simulink model "ACC_CC_model_best_2017aV1"  (Simulink 9.0)
settings: Solver=FixedStepAuto  StartTime=0.0  StopTime=1000  RelTol=1e-3
InitFcn:
  | step=0.001;%时间步长
  | run par.m
values from neighbouring files (symbols this model uses):
  ax_1 = Pop(i,1)    [IGPSO.m]
  ax_2 = Pop(i,2)    [IGPSO.m]
  ess_init_soc = 0.9    [IGPSO.m]
  ess_max_ah_cap = 5    [IGPSO.m]
  ess_r_chg = [0.001393 0.001393 0.001393 0.001393 0.001256 0.001172 0.001099 0.001074 0.001058 0.001066 0.0011 0.001161 0.001244 0.001327 0.001327]*3/5*32    [IGPSO.m]
  ess_r_dis = [0.004178 0.004178 0.004178 0.004178 0.003769 0.003517 0.003296 0.003222 0.003173 0.003197 0.0033 0.003483 0.003732 0.00398 0.00398]*3/5*32    [IGPSO.m]
  ess_soc = [0 0.2 0.25 0.3 0.35 0.4 0.45 0.5 0.55 0.6 0.65 0.7 0.75 0.8 1]    [IGPSO.m]
  ess_voc = [3.124 3.36 3.42 3.479 3.501 3.524 3.547 3.569 3.593 3.616 3.65 3.684 3.72 3.756 3.9]*3*32    [IGPSO.m]
  mc_eff_map = [0.43,0.49,0.58,0.66,0.73,0.70,0.73,0.66,0.58,0.49,0.43 ... (first row only)    [IGPSO.m]
  mc_map_spd = [0;1000;2000;3000;3500;4000;5000;6000;6500;7000;8000]*(2*pi)/60    [IGPSO.m]
  mc_map_trq = motorMAP(1,2:end)    [IGPSO.m]
  mc_max_trq = [142.2;148.6;146.5;92.4;83.9;71.1;56.9;48.4;43.4;37.7;35.6]    [IGPSO.m]
  v_base = 30    [IGPSO.m]
libraries: simulink x2, Solver_SF x1
(part 2 of 2)

== matlab function ACC-CC切换 ==
  data: d_logic1 output double; d_logic2 output double; u output double; vset input double; vp input double; v input double; d input double; d_des input double; lastmodel input double
function [ d_logic1,d_logic2,u]  = fcn(vset,vp,v,d,d_des,lastmodel)
% u=1：代表ACC   U=2代表CC
vset=vset/3.6;
vp=vp/3.6;
v=v/3.6;

k2=1.2;d1=2;
k1=1.999-1.196*exp(-0.1299*(vset-vp));
d_logic1=d_des+k1/2*(vset-vp)+k2*(v-vset)+d1;

k3=2;
d2=2;
k4=1.25;
d_logic2=d_des+k3*(vset-vp)+k4*(v-vp)+d2;

if vp>vset
    if d<d_des
        u=1;
    elseif (d>=d_des)&&(d<d_logic1)
        u=2;
    elseif (d>=d_logic1)&&(d<d_logic2)
        u=2;
    else
        u=2;
    end
else
    if d<d_des
        u=1;
    elseif (d>=d_des)&&(d<d_logic1)
        u=1;
    elseif (d>=d_logic1)&&(d<d_logic2)
        u=lastmodel;  %过渡区
    else
        u=2;
    end
end
end

== matlab function 液压制动控制/MATLAB Function ==
  data: Tm_F input double; T_fric output double; demand_F input double
function T_fric = fcn(Tm_F, demand_F)
if Tm_F<0
    if demand_F<Tm_F
        T_fric=-(demand_F-Tm_F);  %剩余的由摩擦制动实现
    else
        T_fric=0;  %剩余的由摩擦制动实现
        
    end
else
     T_fric=0;  %剩余的由摩擦制动实现
end

== matlab function PNG策略1 ==
  data: vset output double; ID output double; vbase input double; ax input double; v_real input double; ax2 input double; ID_last input double; vset_last input double
function [ vset,ID]    = fcn(vbase,ax,v_real, ax2,ID_last,vset_last)

if v_real>vbase+5   %开始滑行
    ID=1;
    vset=vset_last+ax2*0.001;
    
elseif v_real<vbase-5
    ID=0;
    vset=ax*0.001+vset_last;
else
    if ID_last>0  %上一时刻滑行
       ID=1;
       vset=vset_last+ax2*0.001;
    else
        ID=0;
        vset=vset_last+ax*0.001;
    end
end


end
